simulink model "Cubesat_Controlled"  (R2016a)
settings: Solver=ode4  StartTime=0.0  StopTime=3000  FixedStep=1  MaxStep=11  MinStep=10  RelTol=1e-3
libraries: aerolibutil x7, aerolibtransform2 x3, simulink_extras x3, dspmtrx3 x1, vrlib x1
settings Model: RequirementInfo="{}  %GIDa_15831613_ce61_43ee_92db_7bd4dcc52000"  Creator=Sherief Nabeeh  LastModifiedBy=Sherief Nabeeh
settings SolverCC: ExtrapolationOrder=3
settings DataIOCC: LimitDataPoints=on
settings DebuggingCC: AllowSymbolicDim=off
settings HardwareCC: ProdWordSize=32  ProdHWDeviceType=Specified
settings ModelReferenceCC: PropagateSignalLabelsOutOfModel=off
settings GRTTargetCC: GeneratePreprocessorConditionals=Use local settings

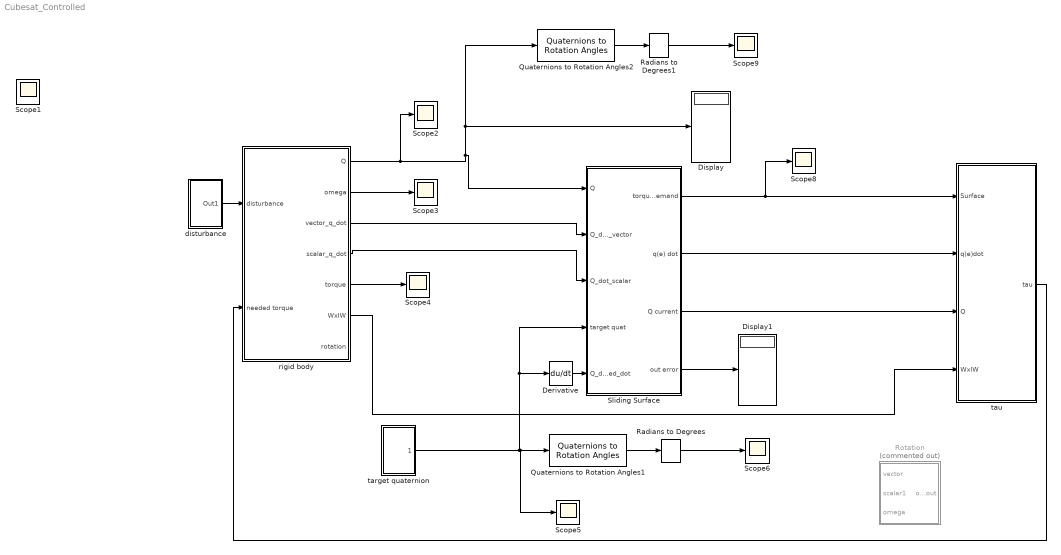
== system Cubesat_Controlled ==
  Derivative : Derivative
  Display : Display
  Display1 : Display
  Quaternions to Rotation Angles1 : aerolibtransform2/Quaternions to Rotation Angles  rotationOrder=ZYX
  Quaternions to Rotation Angles2 : aerolibtransform2/Quaternions to Rotation Angles  rotationOrder=ZYX
  Radians to Degrees : simulink_extras/Transformations/Radians to Degrees
  Radians to Degrees1 : simulink_extras/Transformations/Radians to Degrees
  "Rotation " : Subsystem  Commented=on
  Scope{1..6,8..9} (8 alike) : Scope
  Sliding Surface : Subsystem
  disturbance : Subsystem
  "rigid body " : Subsystem
      settings: ErrorFcn=double
  "target quaternion " : Subsystem
  tau : Subsystem
  wires:
  "rigid body "/2(omega) -> Scope3/1
  "rigid body "/5(torque) -> Scope4/1
  "rigid body "/3(vector_q_dot) -> Sliding Surface/2(Q_dot_vector)
  "rigid body "/4(scalar_q_dot) -> Sliding Surface/3(Q_dot_scalar)
  Derivative/1 -> Sliding Surface/5(Q_desired_dot)
  Quaternions to Rotation Angles1/1 -> Radians to Degrees/1
  Sliding Surface/4(out error) -> Display1/1
  Radians to Degrees/1 -> Scope6/1
  "rigid body "/6(WxIW) -> tau/4(WxIW)
  Sliding Surface/1(torque demand) -> Scope8/1, tau/1(Surface)
  Sliding Surface/2(q(e) dot) -> tau/2(q(e)dot)
  Sliding Surface/3(Q current) -> tau/3(Q)
  "target quaternion "/1(4x1 quat) -> Sliding Surface/4("target quat "), Derivative/1, Scope5/1, Quaternions to Rotation Angles1/1
  disturbance/1(Out1) -> "rigid body "/1(disturbance)
  tau/1(tau) -> "rigid body "/2(needed torque)
  Quaternions to Rotation Angles2/1 -> Radians to Degrees1/1
  Radians to Degrees1/1 -> Scope9/1
  "rigid body "/1("Q ") -> Scope2/1, Sliding Surface/1(Q), Quaternions to Rotation Angles2/1, Display/1

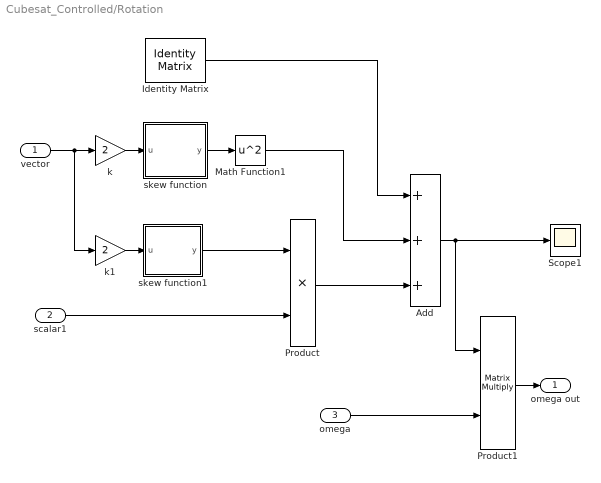
== system Cubesat_Controlled/Rotation  ==
  vector : Inport
  scalar1 : Inport  Port=2
  omega : Inport  Port=3
  Add : Sum  Inputs=+++
  Identity Matrix : dspmtrx3/Identity Matrix  Inherit=off  N=3  Ts=1  dataType=double  isSigned=on  wordLen=16  udDataType=sfix(16)  fracBitsMode=Best precision  numFracBits=15  OutDataTypeStr=double  LastOutDataTypeStr=double
  Math Function1 : Math  Operator=square  SaturateOnIntegerOverflow=on
  Product : Product
  Product1 : Product  Multiplication=Matrix(*)
  Scope1 : Scope
  k : Gain  Gain=2
  k1 : Gain  Gain=2
  skew function : MATLAB Function  TreatAsAtomicUnit=on
  skew function1 : MATLAB Function  TreatAsAtomicUnit=on
  omega out : Outport
  wires:
  vector/1 -> k1/1, k/1
  k/1 -> skew function/1(u)
  k1/1 -> skew function1/1(u)
  skew function1/1(y) -> Product/1
  scalar1/1 -> Product/2
  skew function/1(y) -> Math Function1/1
  Product/1 -> Add/3
  Product1/1 -> omega out/1
  omega/1 -> Product1/2
  Math Function1/1 -> Add/2
  Identity Matrix/1 -> Add/1
  Add/1 -> Scope1/1, Product1/1

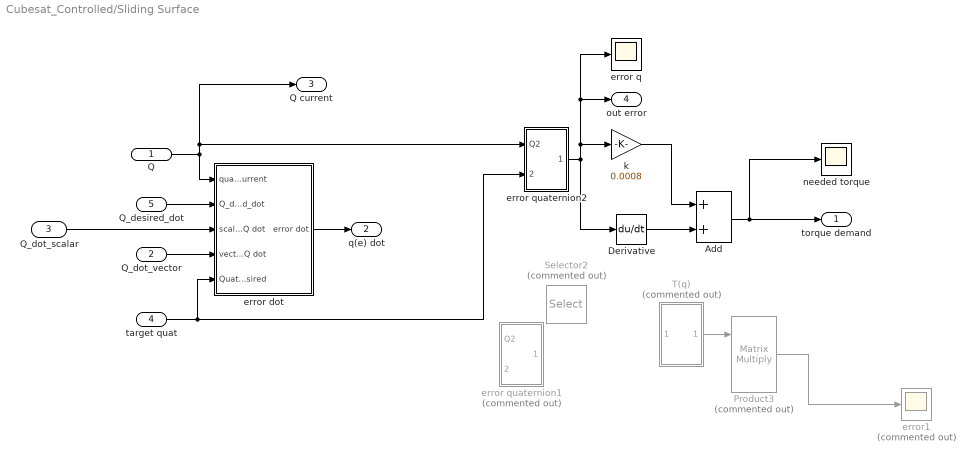
== system Cubesat_Controlled/Sliding Surface ==
  Q : Inport
  Q_dot_vector : Inport  Port=2
  Q_dot_scalar : Inport  Port=3
  "target quat " : Inport  Port=4
  Q_desired_dot : Inport  Port=5
  Add : Sum
  Derivative : Derivative
  Product3 : Product  Commented=on  Multiplication=Matrix(*)
  Selector2 : Selector  Commented=on  InputPortWidth=4  IndexOptions=Index vector (dialog)  Indices=[2,3,4]  OutputSizes=1
  T(q) : Subsystem  Commented=on
  error dot : Subsystem
  error q : Scope
  error quaternion1 : Subsystem  Commented=on
  error quaternion2 : Subsystem
  error1 : Scope  Commented=on
  k : Gain  Gain=0.0008
  needed torque : Scope
  torque demand : Outport
  q(e) dot : Outport  Port=2
  Q current : Outport  Port=3
  out error : Outport  Port=4
  wires:
  Q_dot_scalar/1 -> error dot/3(scalar Q dot)
  Q_dot_vector/1 -> error dot/4(vector Q dot)
  Q_desired_dot/1 -> error dot/2(Q_desired_dot)
  Add/1 -> needed torque/1, torque demand/1
  error dot/1(error dot) -> q(e) dot/1
  k/1 -> Add/1
  Product3/1 -> error1/1
  T(q)/1(Out1) -> Product3/1
  Derivative/1 -> Add/2
  error quaternion2/1(Out1) -> error q/1, out error/1, k/1, Derivative/1
  Q/1 -> error quaternion2/1(Q2), Q current/1, error dot/1("quat current ")
  "target quat "/1 -> error quaternion2/2(In1), error dot/5(Quat desired)

== system Cubesat_Controlled/disturbance ==
  Constant1 : Constant  Value=1e-7
  Constant2 : Constant  Value=1e-7
  Constant3 : Constant  Value=1e-7
  "initial quaternion " : Concatenate  NumInputs=3  Mode=Multidimensional array
  Out1 : Outport
  wires:
  Constant1/1 -> "initial quaternion "/2
  Constant3/1 -> "initial quaternion "/3
  Constant2/1 -> "initial quaternion "/1
  "initial quaternion "/1 -> Out1/1

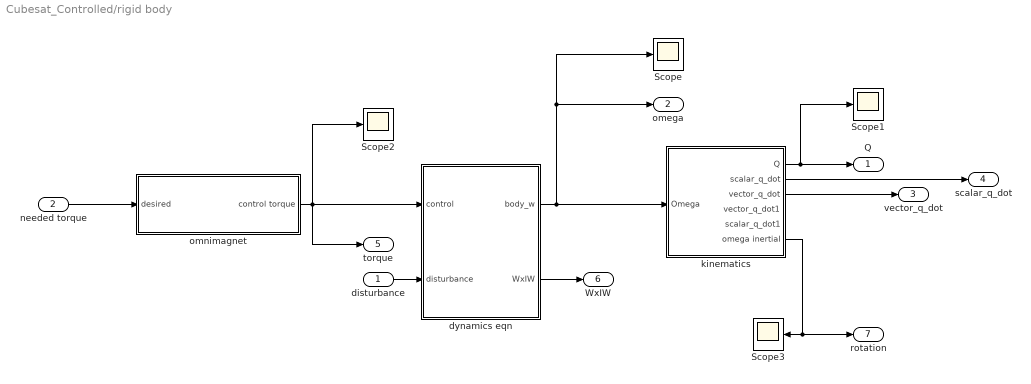
== system Cubesat_Controlled/rigid body  ==
  disturbance : Inport
  needed torque : Inport  Port=2
  Scope{,1..3} (4 alike) : Scope
  dynamics eqn : Subsystem
  kinematics : Subsystem
  omnimagnet : Subsystem
  "Q " : Outport
  omega : Outport  Port=2
  vector_q_dot : Outport  Port=3
  scalar_q_dot : Outport  Port=4
  torque : Outport  Port=5
  WxIW : Outport  Port=6
  rotation : Outport  Port=7
  wires:
  needed torque/1 -> omnimagnet/1(desired)
  omnimagnet/1(control torque) -> Scope2/1, dynamics eqn/1(control), torque/1
  disturbance/1 -> dynamics eqn/2(disturbance)
  kinematics/1(Q) -> Scope1/1, "Q "/1
  kinematics/2(scalar_q_dot) -> scalar_q_dot/1
  dynamics eqn/1(body_w) -> Scope/1, omega/1, kinematics/1(Omega)
  dynamics eqn/2(WxIW) -> WxIW/1
  kinematics/3(vector_q_dot) -> vector_q_dot/1
  kinematics/6(omega inertial) -> Scope3/1, rotation/1

== system Cubesat_Controlled/target quaternion  ==
  Constant : Constant
  Constant1 : Constant  Value=0.15
  Constant2 : Constant  Value=0
  Constant3 : Constant  Value=-0.1
  "initial quaternion " : Concatenate  NumInputs=4  Mode=Multidimensional array
  4x1 quat : Outport
  wires:
  "initial quaternion "/1 -> 4x1 quat/1
  Constant1/1 -> "initial quaternion "/2
  Constant/1 -> "initial quaternion "/1
  Constant2/1 -> "initial quaternion "/3
  Constant3/1 -> "initial quaternion "/4

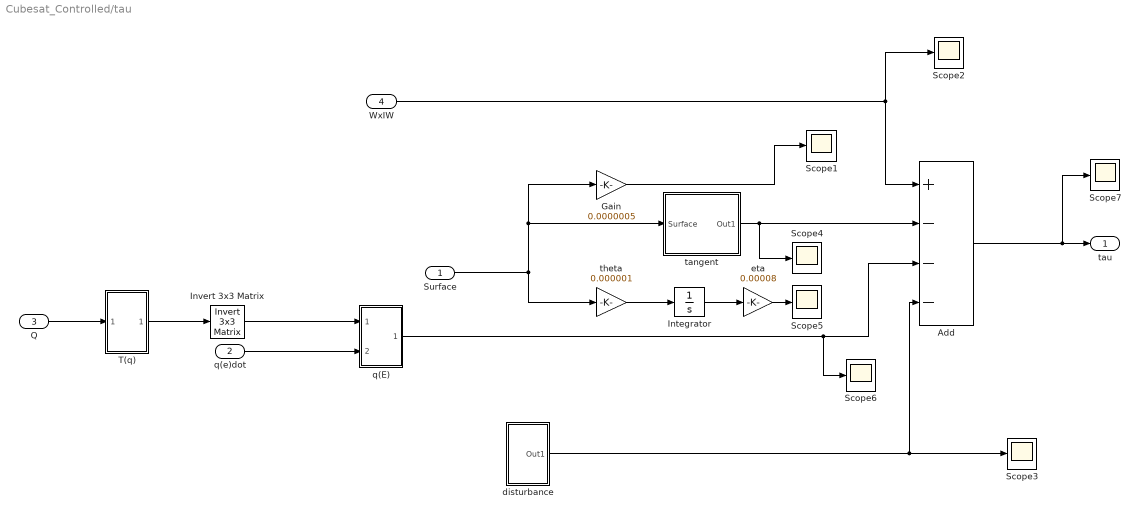
== system Cubesat_Controlled/tau ==
  Surface : Inport
  q(e)dot : Inport  Port=2
  Q : Inport  Port=3
  WxIW : Inport  Port=4
  Add : Sum  Inputs=+---
  Gain : Gain  Gain=0.0000005
  Integrator : Integrator
  Invert 3x3 Matrix : aerolibutil/Invert  3x3 Matrix
  Scope{1..7} (7 alike) : Scope
  T(q) : Subsystem
  disturbance : Subsystem
  eta : Gain  Gain=0.00008
  q(E) : Subsystem
  tangent : Subsystem
  theta : Gain  Gain=0.000001
  tau : Outport
  wires:
  Invert 3x3 Matrix/1 -> q(E)/1(In1)
  Q/1 -> T(q)/1(In1)
  T(q)/1(Out1) -> Invert 3x3 Matrix/1
  Add/1 -> Scope7/1, tau/1
  disturbance/1(Out1) -> Add/4, Scope3/1
  WxIW/1 -> Scope2/1, Add/1
  q(e)dot/1 -> q(E)/2(q(e)dot)
  Surface/1 -> theta/1, Gain/1, tangent/1(Surface)
  tangent/1(Out1) -> Scope4/1, Add/2
  Gain/1 -> Scope1/1
  theta/1 -> Integrator/1
  Integrator/1 -> eta/1
  eta/1 -> Scope5/1
  q(E)/1(Out1) -> Add/3, Scope6/1

== system Cubesat_Controlled/Sliding Surface/T(q) ==
  In1 : Inport
  skew +I+Qt : MATLAB Function  TreatAsAtomicUnit=on
  Out1 : Outport
  wires:
  skew +I+Qt/1(y) -> Out1/1
  In1/1 -> skew +I+Qt/1(u)

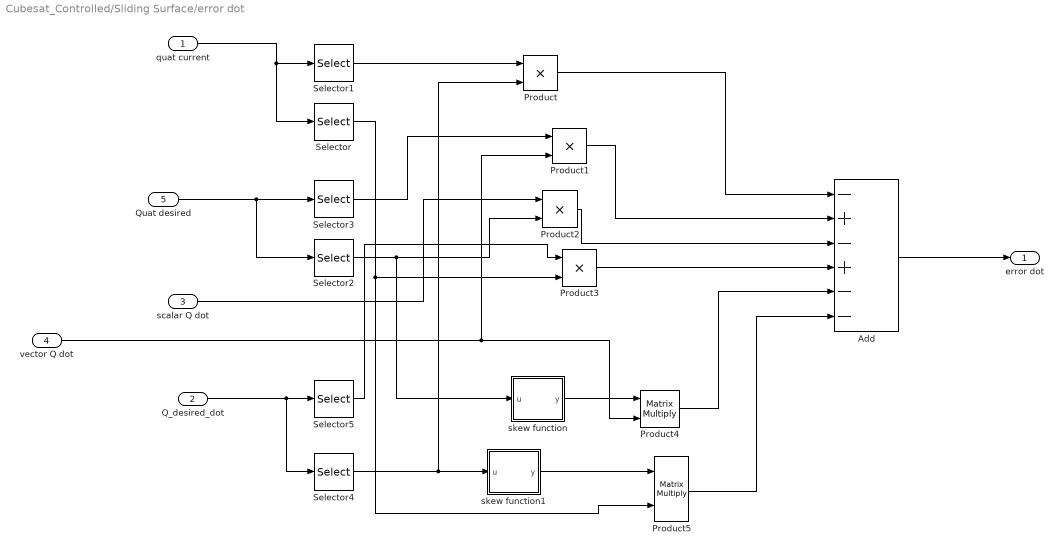
== system Cubesat_Controlled/Sliding Surface/error dot ==
  "quat current " : Inport
  Q_desired_dot : Inport  Port=2
  scalar Q dot : Inport  Port=3
  vector Q dot : Inport  Port=4
  Quat desired : Inport  Port=5
  Add : Sum  Inputs=-+-+--
  Product{,1..3} (4 alike) : Product
  Product4 : Product  Multiplication=Matrix(*)
  Product5 : Product  Multiplication=Matrix(*)
  Selector : Selector  InputPortWidth=4  IndexOptions=Index vector (dialog)  Indices=[2,3,4]  OutputSizes=1
  Selector1 : Selector  InputPortWidth=4  IndexOptions=Index vector (dialog)  Indices=1  OutputSizes=1
  Selector2 : Selector  InputPortWidth=4  IndexOptions=Index vector (dialog)  Indices=[2,3,4]  OutputSizes=1
  Selector3 : Selector  InputPortWidth=4  IndexOptions=Index vector (dialog)  Indices=1  OutputSizes=1
  Selector4 : Selector  InputPortWidth=4  IndexOptions=Index vector (dialog)  Indices=[2,3,4]  OutputSizes=1
  Selector5 : Selector  InputPortWidth=4  IndexOptions=Index vector (dialog)  Indices=1  OutputSizes=1
  skew function : MATLAB Function  TreatAsAtomicUnit=on
  skew function1 : MATLAB Function  TreatAsAtomicUnit=on
  error dot : Outport
  wires:
  "quat current "/1 -> Selector/1, Selector1/1
  Quat desired/1 -> Selector2/1, Selector3/1
  Q_desired_dot/1 -> Selector4/1, Selector5/1
  scalar Q dot/1 -> Product2/1
  vector Q dot/1 -> Product4/2, Product1/2
  Selector1/1 -> Product/1
  Selector4/1 -> Product/2, skew function1/1(u)
  skew function1/1(y) -> Product5/1
  Selector2/1 -> Product2/2, skew function/1(u)
  skew function/1(y) -> Product4/1
  Selector/1 -> Product5/2, Product3/2
  Selector3/1 -> Product1/1
  Selector5/1 -> Product3/1
  Add/1 -> error dot/1
  Product/1 -> Add/1
  Product4/1 -> Add/5
  Product3/1 -> Add/4
  Product2/1 -> Add/3
  Product1/1 -> Add/2
  Product5/1 -> Add/6

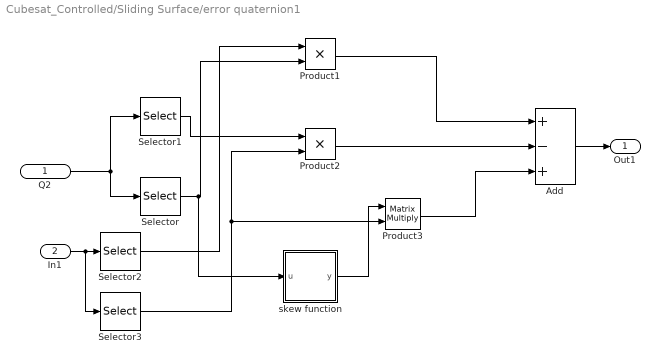
== system Cubesat_Controlled/Sliding Surface/error quaternion1 ==
  Q2 : Inport
  In1 : Inport  Port=2
  Add : Sum  Inputs=+-+
  Product1 : Product
  Product2 : Product
  Product3 : Product  Multiplication=Matrix(*)
  Selector : Selector  InputPortWidth=4  IndexOptions=Index vector (dialog)  Indices=[2,3,4]  OutputSizes=1
  Selector1 : Selector  InputPortWidth=4  IndexOptions=Index vector (dialog)  Indices=1  OutputSizes=1
  Selector2 : Selector  InputPortWidth=4  IndexOptions=Index vector (dialog)  Indices=1  OutputSizes=1
  Selector3 : Selector  InputPortWidth=4  IndexOptions=Index vector (dialog)  Indices=[2,3,4]  OutputSizes=1
  skew function : MATLAB Function  TreatAsAtomicUnit=on
  Out1 : Outport
  wires:
  Product3/1 -> Add/3
  Product2/1 -> Add/2
  Product1/1 -> Add/1
  Selector1/1 -> Product2/1
  Selector/1 -> Product1/2, skew function/1(u)
  Q2/1 -> Selector1/1, Selector/1
  Selector3/1 -> Product2/2, Product3/2
  Selector2/1 -> Product1/1
  In1/1 -> Selector2/1, Selector3/1
  skew function/1(y) -> Product3/1
  Add/1 -> Out1/1

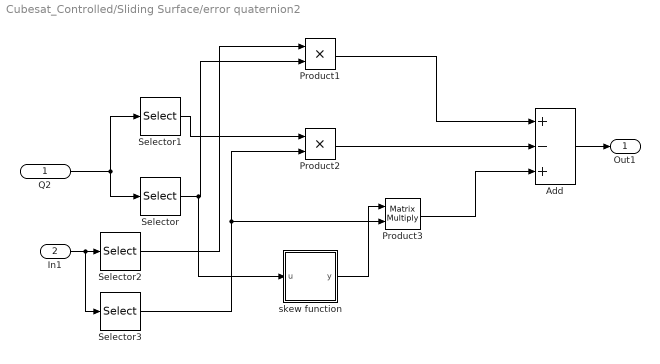
== system Cubesat_Controlled/Sliding Surface/error quaternion2 ==
  Q2 : Inport
  In1 : Inport  Port=2
  Add : Sum  Inputs=+-+
  Product1 : Product
  Product2 : Product
  Product3 : Product  Multiplication=Matrix(*)
  Selector : Selector  InputPortWidth=4  IndexOptions=Index vector (dialog)  Indices=[2,3,4]  OutputSizes=1
  Selector1 : Selector  InputPortWidth=4  IndexOptions=Index vector (dialog)  Indices=1  OutputSizes=1
  Selector2 : Selector  InputPortWidth=4  IndexOptions=Index vector (dialog)  Indices=1  OutputSizes=1
  Selector3 : Selector  InputPortWidth=4  IndexOptions=Index vector (dialog)  Indices=[2,3,4]  OutputSizes=1
  skew function : MATLAB Function  TreatAsAtomicUnit=on
  Out1 : Outport
  wires:
  Add/1 -> Out1/1
  skew function/1(y) -> Product3/1
  In1/1 -> Selector3/1, Selector2/1
  Selector2/1 -> Product1/1
  Selector3/1 -> Product3/2, Product2/2
  Q2/1 -> Selector/1, Selector1/1
  Selector/1 -> skew function/1(u), Product1/2
  Selector1/1 -> Product2/1
  Product1/1 -> Add/1
  Product2/1 -> Add/2
  Product3/1 -> Add/3

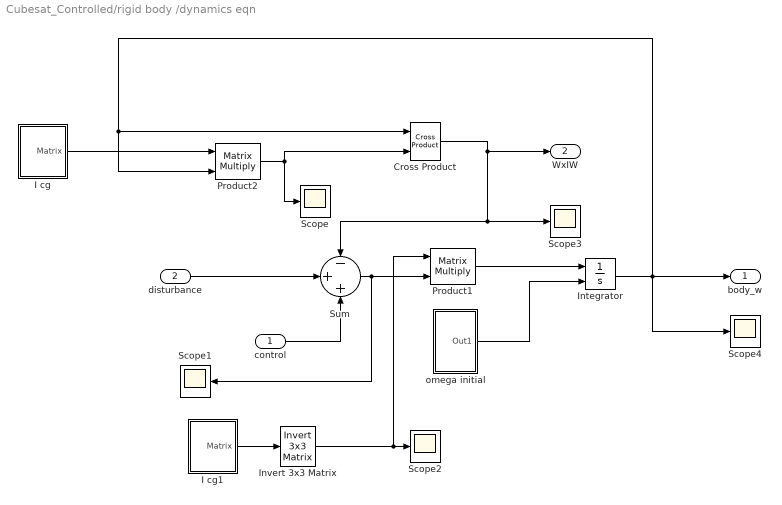
== system Cubesat_Controlled/rigid body /dynamics eqn ==
  control : Inport
  disturbance : Inport  Port=2
  Cross Product : vrlib/Utilities/Cross Product
  I cg : Subsystem
  I cg1 : Subsystem
  Integrator : Integrator  InitialConditionSource=external
  Invert 3x3 Matrix : aerolibutil/Invert  3x3 Matrix
  Product1 : Product  Multiplication=Matrix(*)
  Product2 : Product  Multiplication=Matrix(*)
  Scope{,1..4} (5 alike) : Scope
  Sum : Sum  Inputs=-++
  omega initial : Subsystem
  body_w : Outport
  WxIW : Outport  Port=2
  wires:
  I cg1/1(Matrix) -> Invert 3x3 Matrix/1
  Product1/1 -> Integrator/1
  Cross Product/1 -> Sum/1, Scope3/1, WxIW/1
  disturbance/1 -> Sum/2
  Invert 3x3 Matrix/1 -> Scope2/1, Product1/1
  I cg/1(Matrix) -> Product2/1
  Product2/1 -> Cross Product/2, Scope/1
  omega initial/1(Out1) -> Integrator/2
  Integrator/1 -> Scope4/1, Product2/2, Cross Product/1, body_w/1
  Sum/1 -> Scope1/1, Product1/2
  control/1 -> Sum/3

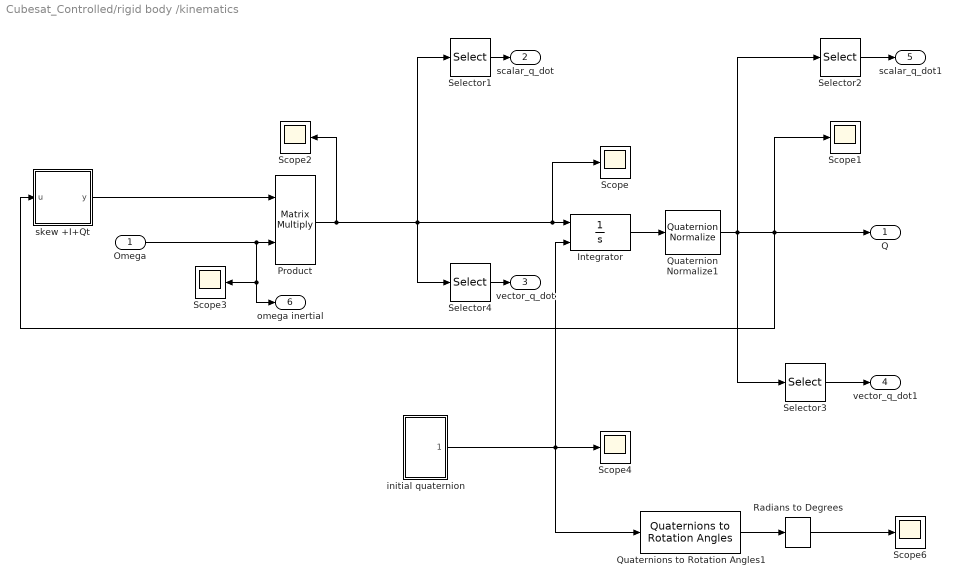
== system Cubesat_Controlled/rigid body /kinematics ==
  Omega : Inport
  Integrator : Integrator  InitialConditionSource=external
  Product : Product  Multiplication=Matrix(*)
  Quaternion Normalize1 : aerolibutil/Quaternion Normalize
  Quaternions to Rotation Angles1 : aerolibtransform2/Quaternions to Rotation Angles  rotationOrder=ZYX
  Radians to Degrees : simulink_extras/Transformations/Radians to Degrees
  Scope{,1..4,6} (6 alike) : Scope
  Selector1 : Selector  InputPortWidth=4  IndexOptions=Index vector (dialog)  Indices=1  OutputSizes=1
  Selector2 : Selector  InputPortWidth=4  IndexOptions=Index vector (dialog)  Indices=1  OutputSizes=1
  Selector3 : Selector  InputPortWidth=4  IndexOptions=Index vector (dialog)  Indices=[2,3,4]  OutputSizes=1
  Selector4 : Selector  InputPortWidth=4  IndexOptions=Index vector (dialog)  Indices=[2,3,4]  OutputSizes=1
  "initial quaternion " : Subsystem
  skew +I+Qt : MATLAB Function  TreatAsAtomicUnit=on
  Q : Outport
  scalar_q_dot : Outport  Port=2
  vector_q_dot : Outport  Port=3
  vector_q_dot1 : Outport  Port=4
  scalar_q_dot1 : Outport  Port=5
  omega inertial : Outport  Port=6
  wires:
  Integrator/1 -> Quaternion Normalize1/1
  Selector4/1 -> vector_q_dot/1
  Selector1/1 -> scalar_q_dot/1
  Omega/1 -> omega inertial/1, Scope3/1, Product/2
  Quaternion Normalize1/1 -> Selector3/1, skew +I+Qt/1(u), Q/1, Scope1/1, Selector2/1
  skew +I+Qt/1(y) -> Product/1
  Product/1 -> Selector4/1, Scope/1, Integrator/1, Selector1/1, Scope2/1
  Selector2/1 -> scalar_q_dot1/1
  Selector3/1 -> vector_q_dot1/1
  "initial quaternion "/1(4x1 quat) -> Quaternions to Rotation Angles1/1, Scope4/1, Integrator/2
  Quaternions to Rotation Angles1/1 -> Radians to Degrees/1
  Radians to Degrees/1 -> Scope6/1

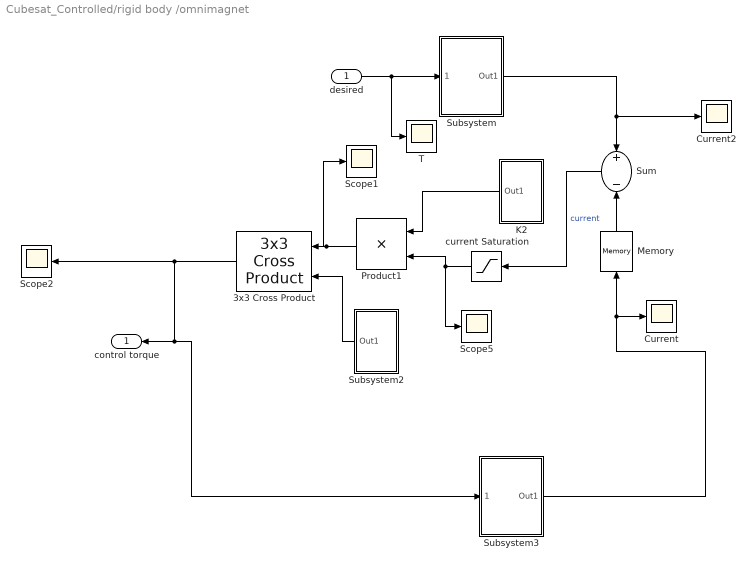
== system Cubesat_Controlled/rigid body /omnimagnet ==
  desired : Inport
  3x3 Cross Product : aerolibutil/3x3 Cross Product
  Current : Scope
  Current2 : Scope
  K2 : Subsystem
  Memory : Memory
  Product1 : Product
  Scope1 : Scope
  Scope2 : Scope
  Scope5 : Scope
  Subsystem : Subsystem
  Subsystem2 : Subsystem
  Subsystem3 : Subsystem
  Sum : Sum  Inputs=+-
  T : Scope
  current Saturation : Saturate  UpperLimit=0.05  LowerLimit=-0.05  LinearizeAsGain=off  ZeroCross=off
  control torque : Outport
  wires:
  Sum/1 -> current Saturation/1  "current"
  Subsystem3/1(Out1) -> Memory/1, Current/1
  Memory/1 -> Sum/2
  Subsystem2/1(Out1) -> 3x3 Cross Product/2
  current Saturation/1 -> Scope5/1, Product1/2
  desired/1 -> T/1, Subsystem/1(desired)
  Subsystem/1(Out1) -> Current2/1, Sum/1
  K2/1(Out1) -> Product1/1
  Product1/1 -> Scope1/1, 3x3 Cross Product/1
  3x3 Cross Product/1 -> Subsystem3/1(desired), control torque/1, Scope2/1

== system Cubesat_Controlled/tau/T(q) ==
  In1 : Inport
  skew +I+Qt : MATLAB Function  TreatAsAtomicUnit=on
  Out1 : Outport
  wires:
  skew +I+Qt/1(y) -> Out1/1
  In1/1 -> skew +I+Qt/1(u)

== system Cubesat_Controlled/tau/disturbance ==
  Constant : Constant  Value=1e-7
  Constant1 : Constant  Value=1e-7
  Constant2 : Constant  Value=1e-7
  "initial quaternion " : Concatenate  NumInputs=3  Mode=Multidimensional array
  Out1 : Outport
  wires:
  Constant1/1 -> "initial quaternion "/2
  Constant2/1 -> "initial quaternion "/3
  Constant/1 -> "initial quaternion "/1
  "initial quaternion "/1 -> Out1/1

== system Cubesat_Controlled/tau/q(E) ==
  In1 : Inport
  q(e)dot : Inport  Port=2
  I cg : Subsystem
  Product1 : Product  Multiplication=Matrix(*)
  Product3 : Product  Multiplication=Matrix(*)
  Scope1 : Scope
  Scope5 : Scope
  k : Gain  Gain=0.0005  Multiplication=Matrix(K*u)
  Out1 : Outport
  wires:
  Product1/1 -> k/1
  k/1 -> Scope5/1, Product3/2
  q(e)dot/1 -> Product1/2
  Product3/1 -> Out1/1, Scope1/1
  I cg/1(Matrix) -> Product1/1
  In1/1 -> Product3/1

== system Cubesat_Controlled/tau/tangent ==
  Surface : Inport
  Divide : Product  Inputs=*/
  Divide1 : Product  Inputs=**
  Scope4 : Scope
  Trigonometric Function : Trigonometry  Operator=tanh
  constant : Constant  Value=0.0005
  constant1 : Constant  Value=3e-5
  Out1 : Outport
  wires:
  Divide/1 -> Trigonometric Function/1
  constant/1 -> Divide/2
  Surface/1 -> Divide/1
  constant1/1 -> Divide1/2
  Trigonometric Function/1 -> Divide1/1
  Divide1/1 -> Out1/1, Scope4/1

== system Cubesat_Controlled/rigid body /dynamics eqn/I cg ==
  Constant : Constant  Value=0.01
  Constant{1..3,5..7} (6 alike) : Constant  Value=0
  Constant4 : Constant  Value=0.01
  Constant8 : Constant  Value=0.01
  Reshape (9) to [3x3] column-major : Reshape  OutputDimensionality=Customize  OutputDimensions=[3,3]
  Vector Concatenate : Concatenate  NumInputs=9
  Matrix : Outport  PortDimensions=[3 3]
  wires:
  Constant4/1 -> Vector Concatenate/5
  Constant5/1 -> Vector Concatenate/6
  Reshape (9) to [3x3] column-major/1 -> Matrix/1
  Constant8/1 -> Vector Concatenate/9
  Constant7/1 -> Vector Concatenate/8
  Constant6/1 -> Vector Concatenate/7
  Constant2/1 -> Vector Concatenate/3
  Constant1/1 -> Vector Concatenate/2
  Constant/1 -> Vector Concatenate/1
  Constant3/1 -> Vector Concatenate/4
  Vector Concatenate/1 -> Reshape (9) to [3x3] column-major/1

== system Cubesat_Controlled/rigid body /dynamics eqn/I cg1 ==
  Constant : Constant  Value=0.01
  Constant{1..3,5..7} (6 alike) : Constant  Value=0
  Constant4 : Constant  Value=0.01
  Constant8 : Constant  Value=0.01
  Reshape (9) to [3x3] column-major : Reshape  OutputDimensionality=Customize  OutputDimensions=[3,3]
  Vector Concatenate : Concatenate  NumInputs=9
  Matrix : Outport  PortDimensions=[3 3]
  wires:
  Vector Concatenate/1 -> Reshape (9) to [3x3] column-major/1
  Constant3/1 -> Vector Concatenate/4
  Constant/1 -> Vector Concatenate/1
  Constant1/1 -> Vector Concatenate/2
  Constant2/1 -> Vector Concatenate/3
  Constant6/1 -> Vector Concatenate/7
  Constant7/1 -> Vector Concatenate/8
  Constant8/1 -> Vector Concatenate/9
  Reshape (9) to [3x3] column-major/1 -> Matrix/1
  Constant5/1 -> Vector Concatenate/6
  Constant4/1 -> Vector Concatenate/5

== system Cubesat_Controlled/rigid body /dynamics eqn/omega initial ==
  Constant : Constant  Value=0.001
  Constant1 : Constant  Value=0.001
  Constant2 : Constant  Value=0.001
  "initial quaternion " : Concatenate  NumInputs=3
  Out1 : Outport
  wires:
  Constant1/1 -> "initial quaternion "/2
  Constant2/1 -> "initial quaternion "/3
  Constant/1 -> "initial quaternion "/1
  "initial quaternion "/1 -> Out1/1

== system Cubesat_Controlled/rigid body /kinematics/initial quaternion  ==
  Constant : Constant
  Constant1 : Constant  Value=0
  Constant2 : Constant  Value=0
  Constant3 : Constant  Value=0
  "initial quaternion " : Concatenate  NumInputs=4  Mode=Multidimensional array
  4x1 quat : Outport
  wires:
  "initial quaternion "/1 -> 4x1 quat/1
  Constant1/1 -> "initial quaternion "/2
  Constant/1 -> "initial quaternion "/1
  Constant2/1 -> "initial quaternion "/3
  Constant3/1 -> "initial quaternion "/4

== system Cubesat_Controlled/rigid body /omnimagnet/K2 ==
  Constant : Constant  Value=0.5
  Constant1 : Constant  Value=0.5
  Constant2 : Constant  Value=0.5
  Vector Concatenate : Concatenate  NumInputs=3  Mode=Multidimensional array
  Out1 : Outport
  wires:
  Constant1/1 -> Vector Concatenate/2
  Constant2/1 -> Vector Concatenate/3
  Constant/1 -> Vector Concatenate/1
  Vector Concatenate/1 -> Out1/1

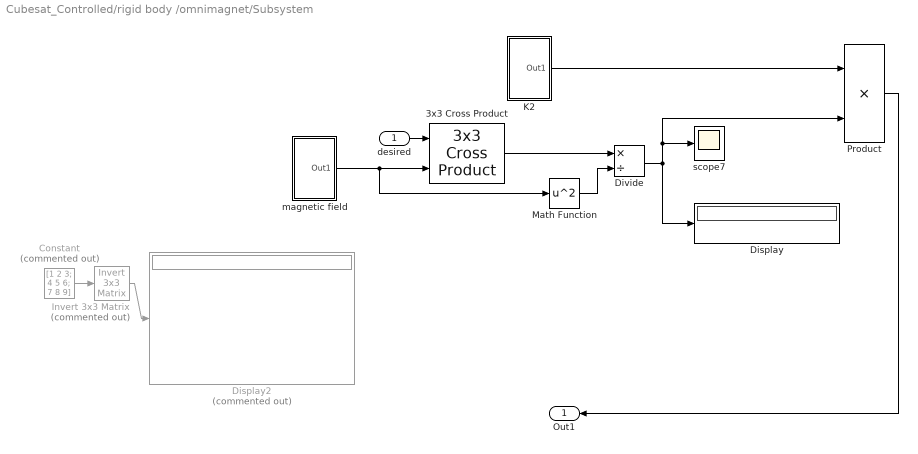
== system Cubesat_Controlled/rigid body /omnimagnet/Subsystem ==
  desired : Inport
  3x3 Cross Product : aerolibutil/3x3 Cross Product
  Constant : Constant  Commented=on  Value=[1 2 3; 4 5 6; 7 8 9]
  Display : Display
  Display2 : Display  Commented=on
  Divide : Product  Inputs=*/
  Invert 3x3 Matrix : aerolibutil/Invert  3x3 Matrix  Commented=on
  K2 : Subsystem
  Math Function : Math  Operator=square  SaturateOnIntegerOverflow=on
  Product : Product
  magnetic field : Subsystem
  scope7 : Scope
  Out1 : Outport
  wires:
  Product/1 -> Out1/1
  Divide/1 -> Display/1, scope7/1, Product/2
  magnetic field/1(Out1) -> Math Function/1, 3x3 Cross Product/2
  K2/1(Out1) -> Product/1
  Constant/1 -> Invert 3x3 Matrix/1
  Invert 3x3 Matrix/1 -> Display2/1
  desired/1 -> 3x3 Cross Product/1
  3x3 Cross Product/1 -> Divide/1
  Math Function/1 -> Divide/2

== system Cubesat_Controlled/rigid body /omnimagnet/Subsystem2 ==
  Constant : Constant  Value=0.00005
  Constant1 : Constant  Value=0.00005
  Constant2 : Constant  Value=0.00005
  Vector Concatenate : Concatenate  NumInputs=3  Mode=Multidimensional array
  Out1 : Outport
  wires:
  Vector Concatenate/1 -> Out1/1
  Constant/1 -> Vector Concatenate/1
  Constant2/1 -> Vector Concatenate/3
  Constant1/1 -> Vector Concatenate/2

== system Cubesat_Controlled/rigid body /omnimagnet/Subsystem3 ==
  desired : Inport
  3x3 Cross Product : aerolibutil/3x3 Cross Product
  Current1 : Scope
  K2 : Subsystem
  Product : Product
  magnetic field : Subsystem
  Out1 : Outport
  wires:
  K2/1(Out1) -> Product/1
  magnetic field/1(Out1) -> 3x3 Cross Product/2
  desired/1 -> 3x3 Cross Product/1
  3x3 Cross Product/1 -> Product/2, Current1/1
  Product/1 -> Out1/1

== system Cubesat_Controlled/tau/q(E)/I cg ==
  Constant : Constant  Value=0.001
  Constant{1..3,5..7} (6 alike) : Constant  Value=0
  Constant4 : Constant  Value=0.001
  Constant8 : Constant  Value=0.001
  Reshape (9) to [3x3] column-major : Reshape  OutputDimensionality=Customize  OutputDimensions=[3,3]
  Vector Concatenate : Concatenate  NumInputs=9
  Matrix : Outport  PortDimensions=[3 3]
  wires:
  Constant4/1 -> Vector Concatenate/5
  Constant5/1 -> Vector Concatenate/6
  Reshape (9) to [3x3] column-major/1 -> Matrix/1
  Constant8/1 -> Vector Concatenate/9
  Constant7/1 -> Vector Concatenate/8
  Constant6/1 -> Vector Concatenate/7
  Constant2/1 -> Vector Concatenate/3
  Constant1/1 -> Vector Concatenate/2
  Constant/1 -> Vector Concatenate/1
  Constant3/1 -> Vector Concatenate/4
  Vector Concatenate/1 -> Reshape (9) to [3x3] column-major/1

== system Cubesat_Controlled/rigid body /omnimagnet/Subsystem/K2 ==
  Constant : Constant  Value=2
  Constant1 : Constant  Value=2
  Constant2 : Constant  Value=2
  Vector Concatenate : Concatenate  NumInputs=3  Mode=Multidimensional array
  Out1 : Outport
  wires:
  Constant1/1 -> Vector Concatenate/2
  Constant2/1 -> Vector Concatenate/3
  Constant/1 -> Vector Concatenate/1
  Vector Concatenate/1 -> Out1/1

== system Cubesat_Controlled/rigid body /omnimagnet/Subsystem/magnetic field ==
  Clock : Clock
  Clock1 : Clock
  Clock2 : Clock
  Constant : Constant  Value=9^-5
  Constant1 : Constant  Value=10^-5
  Constant2 : Constant  Value=11^-5
  Sine Wave Function1 : Sin  TimeSource=Use external signal  Amplitude=9e-5  Frequency=25  Phase=4  SampleTime=0  VectorParams1D=off  Offset=100
  Sine Wave Function2 : Sin  TimeSource=Use external signal  Amplitude=9e-5  Frequency=25  Phase=4  SampleTime=0  VectorParams1D=off  Offset=100
  Sine Wave Function3 : Sin  TimeSource=Use external signal  Amplitude=9e-5  Frequency=25  Phase=4  SampleTime=0  VectorParams1D=off  Offset=100
  Vector Concatenate : Concatenate  NumInputs=3  Mode=Multidimensional array
  Vector Concatenate1 : Concatenate  NumInputs=3  Mode=Multidimensional array
  Out1 : Outport
  wires:
  Constant/1 -> Vector Concatenate/1
  Constant2/1 -> Vector Concatenate/3
  Constant1/1 -> Vector Concatenate/2
  Sine Wave Function1/1 -> Vector Concatenate1/2
  Vector Concatenate1/1 -> ?
  Sine Wave Function2/1 -> Vector Concatenate1/1
  Sine Wave Function3/1 -> Vector Concatenate1/3
  Clock/1 -> Sine Wave Function2/1
  Clock1/1 -> Sine Wave Function1/1
  Clock2/1 -> Sine Wave Function3/1
  Vector Concatenate/1 -> Out1/1

== system Cubesat_Controlled/rigid body /omnimagnet/Subsystem3/K2 ==
  Constant : Constant  Value=1/6000
  Constant1 : Constant  Value=1/6000
  Constant2 : Constant  Value=1/6000
  Vector Concatenate : Concatenate  NumInputs=3  Mode=Multidimensional array
  Out1 : Outport
  wires:
  Vector Concatenate/1 -> Out1/1
  Constant/1 -> Vector Concatenate/1
  Constant2/1 -> Vector Concatenate/3
  Constant1/1 -> Vector Concatenate/2

== system Cubesat_Controlled/rigid body /omnimagnet/Subsystem3/magnetic field ==
  Constant : Constant  Value=0.00005
  Constant1 : Constant  Value=0.00005
  Constant2 : Constant  Value=0.00005
  Vector Concatenate : Concatenate  NumInputs=3  Mode=Multidimensional array
  Out1 : Outport
  wires:
  Constant1/1 -> Vector Concatenate/2
  Constant2/1 -> Vector Concatenate/3
  Constant/1 -> Vector Concatenate/1
  Vector Concatenate/1 -> Out1/1

== matlab function Cubesat_Controlled/Rotation /skew function ==
  data: u input; y output
function y = fcn(u)
%#codegen
y = [0 -u(3) u(2) ; u(3) 0 -u(1); -u(2) u(1) 0] ;

== matlab function Cubesat_Controlled/rigid body /kinematics/skew +I+Qt ==
  data: u input; y output
function y = fcn(u)
%#codegen
y = [u(1) -u(4) u(3) ; u(4) u(1) -u(2); -u(3) u(2) u(1);-u(2) -u(3) -u(4)] ;

== matlab function Cubesat_Controlled/Sliding Surface/error dot/skew function ==
  data: u input; y output
function y = fcn(u)
%#codegen
y = [0 -u(3) u(2) ; u(3) 0 -u(1); -u(2) u(1) 0] ;

== matlab function Cubesat_Controlled/tau/T(q)/skew +I+Qt ==
  data: u input; y output
function y = fcn(u)
%#codegen
y = [u(1) -u(4) u(3) ; u(4) u(1) -u(2); -u(3) u(2) u(1)] ;

== matlab function Cubesat_Controlled/Sliding Surface/T(q)/skew +I+Qt ==
  data: u input; y output
function y = fcn(u)
%#codegen
y = [u(1) -u(4) u(3) ; u(4) u(1) -u(2); -u(3) u(2) u(1)] ;

== matlab function Cubesat_Controlled/Sliding Surface/error quaternion1/skew function ==
  data: u input; y output
function y = fcn(u)
%#codegen
y = [0 -u(3) u(2) ; u(3) 0 -u(1); -u(2) u(1) 0] ;

== matlab function Cubesat_Controlled/Sliding Surface/error quaternion2/skew function ==
  data: u input; y output
function y = fcn(u)
%#codegen
y = [0 -u(3) u(2) ; u(3) 0 -u(1); -u(2) u(1) 0] ;

== matlab function Cubesat_Controlled/Rotation /skew function1 ==
  data: u input; y output
function y = fcn(u)
%#codegen
y = [0 -u(3) u(2) ; u(3) 0 -u(1); -u(2) u(1) 0] ;

== matlab function Cubesat_Controlled/Sliding Surface/error dot/skew function1 ==
  data: u input; y output
function y = fcn(u)
%#codegen
y = [0 -u(3) u(2) ; u(3) 0 -u(1); -u(2) u(1) 0] ;
